simulink model "untitled"  (R2021a)
settings: Solver=VariableStepAuto  StartTime=0.0  StopTime=10.0  RelTol=1e-3
settings Model: Creator=sophi  LastModifiedBy=sophi

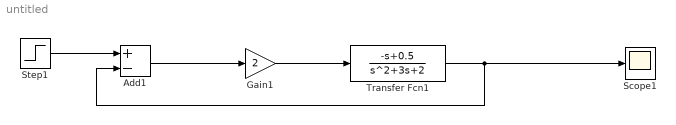
== system untitled ==
  Add1 : Sum  Inputs=+-
  Gain1 : Gain  Gain=2
  Scope1 : Scope
  Step1 : Step  After=10  SampleTime=0
  Transfer Fcn1 : TransferFcn  Numerator=[-1 0.5]  Denominator=[1 3 2]
  wires:
  Step1/1 -> Add1/1
  Add1/1 -> Gain1/1
  Gain1/1 -> Transfer Fcn1/1
  Transfer Fcn1/1 -> Scope1/1, Add1/2
